simulink model "VSC"  (R2023a)
settings: Solver=FixedStepAuto  StartTime=0.0  StopTime=1  FixedStep=2e-6  RelTol=1e-3
InitFcn:
  | Ts=2e-6;
  | idref=20;
  | iqref=0;
  | Rs=3.75;
  | Ls=12e-3;
  | Lc=1.5e-3;
  | Us=100*sqrt(2);
  | omega_gn = 100*pi;
  | delta_ss=asin((omega_gn*Ls*idref+Rs*iqref)/Us);
  | zeta=0.5;
  | ts=0.1;
  | Kp=18.4/Us/ts;
  | Ki=43.32/Us/(zeta*ts)^2;
  | beta = 10*pi;
  | 
  | % Fault-time voltage dip
  | deltaV = 38.94*sqrt(2);
  | 
  | % Anti-windup parameters
  | k1=0;
  | k2=0;
  | % k1 = 5.9289;
  | % k2 = -7.7758;
  | % k2 = -k1 * Kp;
  | 
  | % performance-based activation of AW
  | % F = -353.46;
  | % F = -208.55;
  | F = 0;
undefined symbols (not defined in the file): Gp, Gq
libraries: spsControlledVoltageSourceLib x6, spsGroundLib x3, spsThreePhaseSeriesRLCBranchLib x3, eeGeneralControl x2, spsabctodq0Lib x2, spsPower3phInstantaneousLib x1, spsThreePhaseVIMeasurementLib x1, spsdq0toabcLib x1, spspowerguiLib x1
settings Model: Creator=Dell  LastModifiedBy=John Jackal
settings OptimizationCC: ReuseModelBlockBuffer=off
settings ModelReferenceCC: EnableRefExpFcnMdlSchedulingChecks=on

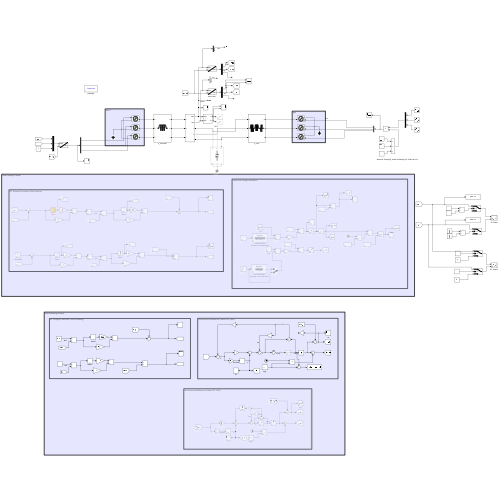
[thumbnail: Simulink's stored preview of the top-level diagram]
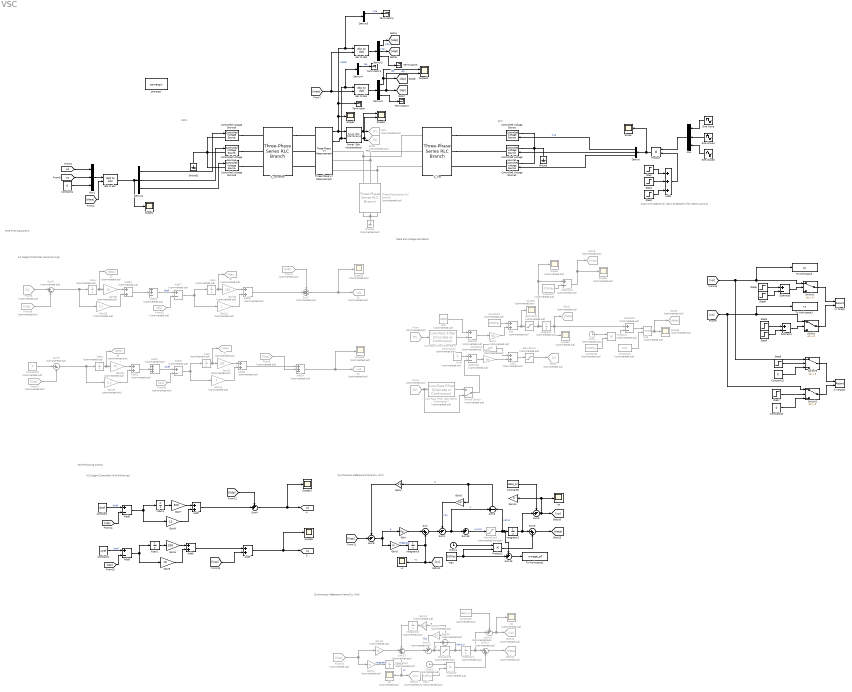
== system VSC ==
  note: Grid-Following Control
  note: Grid-Froming Control
  note: Synchronous-Reference Frame PLL (AW)
  note: AC Subgrid Controller (Grid-Following)
  note: PCC
  note: theta and voltage calculation
  note: start with 100sqrt(2), down to 60sqrt(2) for 100ms at t=1s
  note: grid
  note: VSC1
  note: AC Subgrid Controller (Grid-Forming)
  note: Synchronous-Reference Frame PLL (AW)
  "   21" : Goto  Commented=on  GotoTag=Xqaci  TagVisibility=global
  "   22" : Goto  Commented=on  GotoTag=Xdaci  TagVisibility=global
  "   23" : Goto  Commented=on  GotoTag=vq1  TagVisibility=global
  "   24" : Goto  Commented=on  GotoTag=vd1  TagVisibility=global
  "   25" : Goto  Commented=on  GotoTag=Xdacv  TagVisibility=global
  "   28" : Goto  Commented=on  GotoTag=Xqacv  TagVisibility=global
  Add{,1,22..23,25..26} (6 alike) : Sum  Commented=on
  Add19 : Sum  Commented=on  Inputs=++-
  Add2 : Sum  Inputs=+++
  Add21 : Sum  Commented=on  Inputs=+++
  Add24 : Sum  Commented=on  Inputs=++-
  Add27 : Sum  Commented=on  Inputs=+-
  Add28 : Sum  Commented=on  Inputs=+-
  Add5 : Sum
  Add6 : Sum
  Add7 : Sum
  Add8 : Sum  Inputs=+-
  Add9 : Sum  Inputs=+-
  Clock : Clock  Commented=on
  Clock1 : Clock
  Clock2 : Clock  Commented=on
  Constant : Constant  Value=idref
  Constant1 : Constant  Commented=on  Value=2*50*pi
  Constant10 : Constant  Value=0
  Constant11 : Constant  Value=0
  Constant2 : Constant  Value=iqref
  Constant20 : Constant  Commented=on  Value=0
  Constant3 : Constant  Commented=on  Value=100
  Constant4 : Constant  Value=0
  Constant5 : Constant  Commented=on  Value=2*50*pi
  Constant6 : Constant  Commented=on  Value=2*pi
  Constant7 : Constant  Commented=on  Value=2*50*pi
  Constant8 : Constant  Value=delta_ss
  Constant9 : Constant  Commented=on  Value=delta_ss
  Controlled Voltage Source{,1..5} (6 alike) : spsControlledVoltageSourceLib/Controlled Voltage Source  Initialize=on  Source_Type=AC  Amplitude=0  Phase=0  Frequency=0  Measurements=None
  Demux{,1..5} (6 alike) : Demux  Outputs=3
  From : From  Commented=on  GotoTag=P
  From1 : From  Commented=on  GotoTag=Q
  From16 : From  Commented=on  GotoTag=Uqp
  From39 : From  Commented=on  GotoTag=Uds
  From4 : From  Commented=on  GotoTag=Uds
  From47 : From  Commented=on  GotoTag=Uqs
  From5 : From  Commented=on  GotoTag=Uqs
  From6 : From  Commented=on  GotoTag=V
  From62 : From  Commented=on  GotoTag=ids
  From63 : From  Commented=on  GotoTag=iqs
  Gain : Gain  Gain=Kp
  Gain1 : Gain  Commented=on  Gain=Gp
  Gain10 : Gain  Commented=on  Gain=Kp
  Gain11 : Gain  Commented=on  Gain=Ki
  Gain12 : Gain  Commented=on  Gain=k1
  Gain13 : Gain  Commented=on  Gain=k2
  Gain14 : Gain  Gain=F
  Gain2 : Gain  Commented=on  Gain=Gq
  Gain29 : Gain  Commented=on  Gain=100
  Gain3 : Gain  Gain=Ki
  Gain30 : Gain  Commented=on  Gain=100
  Gain31 : Gain  Commented=on
  Gain35 : Gain  Commented=on  Gain=0.1
  Gain36 : Gain  Commented=on  Gain=10
  Gain37 : Gain  Commented=on  Gain=0.1
  Gain39 : Gain  Commented=on  Gain=10
  Gain4 : Gain  Gain=k1
  Gain41 : Gain  Commented=on
  Gain5 : Gain  Gain=k2
  Gain6 : Gain  Gain=500
  Gain7 : Gain  Gain=500
  Gain8 : Gain  Gain=10
  Gain9 : Gain  Gain=10
  Goto : Goto  Commented=on  GotoTag=P
  Goto1 : Goto  Commented=on  GotoTag=Q
  Goto12 : Goto  Commented=on  GotoTag=xp
  Goto14 : Goto  Commented=on  GotoTag=xc
  Goto15 : Goto  Commented=on  GotoTag=theta
  Goto2 : Goto  Commented=on  GotoTag=theta
  Goto3 : Goto  Commented=on  GotoTag=V
  Goto8 : Goto  Commented=on  GotoTag=delta
  Goto9 : Goto  Commented=on  GotoTag=omega
  Ground : spsGroundLib/Ground  LConnTagsString=a
  Ground1 : spsGroundLib/Ground  Commented=on  LConnTagsString=a
  Ground2 : spsGroundLib/Ground  LConnTagsString=a
  Integrator{,1,3..4} (4 alike) : Integrator  Commented=on
  Integrator2 : Integrator
  Integrator5 : Integrator
  Low-Pass Filter (Discrete or Continuous) : eeGeneralControl/Low-Pass Filter (Discrete or Continuous)  Commented=on  K=1  T=1/(2*pi*50)  B=inf  A=-inf  init_option=Inherited from block input  x0=0  Ts=-1
  Low-Pass Filter (Discrete or Continuous)1 : eeGeneralControl/Low-Pass Filter (Discrete or Continuous)  Commented=on  K=1  T=1/(2*pi*0.1)  B=inf  A=-inf  init_option=Inherited from block input  x0=0  Ts=-1
  Manual Switch : ManualSwitch  Commented=on  CurrentSetting=0
  Mod : Math  Commented=on  Operator=mod
  Mux : Mux  Inputs=3
  Mux1 : Mux  Inputs=3
  "Power (3ph, Instantaneous)" : spsPower3phInstantaneousLib/Power (3ph, Instantaneous)
  Pref : Constant  Commented=on  Value=2000
  Product : Product
  Product1 : Product  Commented=on
  Product2 : Product
  Product3 : Product  Commented=on
  Qref : Constant  Commented=on  Value=0
  Saturation : Saturate  Commented=on  UpperLimit=51*2*pi  LowerLimit=49*2*pi
  Saturation1 : Saturate  Commented=on  UpperLimit=150  LowerLimit=50
  Saturation2 : Saturate  Commented=through  UpperLimit=beta  LowerLimit=-beta
  Saturation3 : Saturate  Commented=on  UpperLimit=10*pi  LowerLimit=-10*pi
  Scope{,1..2,9..10} (5 alike) : Scope
  Scope11 : Scope  NumInputPorts=2
  Scope{4..8,18,25} (7 alike) : Scope  Commented=on
  Scope3 : Scope  NumInputPorts=2
  Sine Wave : Sin  Frequency=50*2*pi  SampleTime=Ts
  Sine Wave1 : Sin  Frequency=50*2*pi  Phase=-2/3*pi  SampleTime=Ts
  Sine Wave2 : Sin  Frequency=50*2*pi  Phase=2/3*pi  SampleTime=Ts
  Step : Step  Time=0  Before=Us  After=Us  SampleTime=0
  Step1 : Step  Time=0.1  After=-deltaV  SampleTime=0
  Step2 : Step  Time=0.2  After=deltaV  SampleTime=0
  Step3 : Step  Time=0  SampleTime=0
  Step4 : Step  SampleTime=0
  Step5 : Step  Time=0  SampleTime=0
  Step6 : Step  SampleTime=0
  Step7 : Step  Time=3  SampleTime=0
  Step9 : Step  Time=3  SampleTime=0
  Subtract{,1..3} (4 alike) : Sum  Commented=on  Inputs=+-
  Subtract4 : Sum  Inputs=+-
  Subtract5 : Sum  Inputs=+-
  Sum : Sum  Inputs=|++
  Sum1 : Sum  Inputs=-+|
  Sum10 : Sum  Commented=on  Inputs=-++
  Sum11 : Sum  Commented=on  Inputs=-+|
  Sum12 : Sum  Commented=on  Inputs=+-
  Sum13 : Sum  Commented=on  Inputs=|++
  Sum14 : Sum  Commented=on  Inputs=-+|
  Sum15 : Sum  Inputs=++|
  Sum16 : Sum  Inputs=++|
  Sum2 : Sum  Inputs=+-
  Sum3 : Sum  Inputs=|++
  Sum4 : Sum  Inputs=++|
  Sum5 : Sum  Inputs=-+|
  Sum6 : Sum  Commented=on  Inputs=|+-
  Sum7 : Sum  Commented=on  Inputs=+++
  Sum8 : Sum  Inputs=-+|
  Sum9 : Sum  Commented=on  Inputs=|+-
  Switch{,1..3} (4 alike) : Switch  Criteria=u2 > Threshold  SaturateOnIntegerOverflow=off  InputSameDT=off
  Terminator{,1..4} (5 alike) : Terminator
  Three-Phase Series RLC Branch1 : spsThreePhaseSeriesRLCBranchLib/Three-Phase Series RLC Branch  Commented=on  LConnTagsString=A|B|C  RConnTagsString=A|B|C  BranchType=C  Resistance=1  Inductance=1e-3  Capacitance=20e-6  Measurements=None
  Three-Phase V-I Measurement : spsThreePhaseVIMeasurementLib/Three-Phase V-I Measurement  VoltageMeasurement=phase-to-ground  SetLabelV=off  LabelV=Vabc  Vpu=off  VpuLL=off  CurrentMeasurement=yes  SetLabelI=off  LabelI=Iabc  Ipu=off  Pbase=100e6  Vbase=500e3  OutputType=Complex  PhasorSimulation=off  PSBequivalent=0
  To Workspace : ToWorkspace  VariableName=xp  SampleTime=-1
  To Workspace1 : ToWorkspace  VariableName=xc  SampleTime=-1
  To Workspace2 : ToWorkspace  VariableName=omega_pll  SampleTime=-1
  XY Graph : Record  RecordToWorkspace=on  FileSettingsInternal="{\"entries\":[{\"content\":{\"excelSettings\":{\"content\":{},\"type\":\"Streamout.ExcelSettings\"}},\"type\":\"Streamout.FileSettingStorage\",\"uuid\":\"61cb4bfb-05d6-417b-9b14-40baebda5446\"}],\"packageUris\":[\"http://schema.mathworks.com/mf0/streamout_blocks/R2020a\"],\"version\":\"1.0\"}"  Layout=[1 1]  SignalsInternal="{\"entries\":[{\"content\":{\"signals\":[{\"content\":{\"blockPath\":[\"VSC/XY Graph\"],\"dimensions\":[1],\"domain\":\"VSC/XY Graph\",\"lineColor\":\"#a2142f\",\"plots\":[1],\"port\":1,\"sid\":[\"\"],\"signalID\":410486,\"signalName\":\"Switch1\"},\"type\":\"RecordBlkView.Signal\",\"uuid\":\"486c21a0-9f22-4725-bac4-aafadb3d172d\"},{\"content\":{\"blockPath\":[\"VSC/XY Graph\"],\"dimensions\":[1],\"domain\":\"VSC/XY Graph\",\"lineColor\":\"#139fff\",\"plots\":[1],\"port\":2,\"sid\":[\"\"],\"signalID\":410490,\"signalName\":\"Switch\"},\"type\":\"RecordBlkView.Signal\",\"uuid\":\"b45c9456-2913-48ec-872b-2d38d1e96725\"}]},\"type\":\"RecordBlkView.InputSignals\",\"uuid\":\"3a20c26a-c753-4ebd-9899-0a237facdabc\"}],\"packageUris\":[\"http://schema.mathworks.com/mf0/streamout_blocks/R2020a\"],\"version\":\"1.0\"}"  VisualizationBindings="{\"xyplotplugin\":{\"info\":[{\"series\":[{\"bindingParametersList\":[{\"parameter\":\"X-Axis\",\"signalID\":410486,\"signalName\":\"Switch1\"},{\"parameter\":\"Y-Axis\",\"signalID\":410490,\"signalName\":\"Switch\"}],\"seriesID\":23615}],\"subplotID\":1}]}}"  CompatibilityTag=XY
  XY Graph1 : Record  FileSettingsInternal="{\"entries\":[{\"content\":{\"excelSettings\":{\"content\":{},\"type\":\"Streamout.ExcelSettings\"}},\"type\":\"Streamout.FileSettingStorage\",\"uuid\":\"121f3693-127c-40a0-ad6a-a4d3c19ad6c3\"}],\"packageUris\":[\"http://schema.mathworks.com/mf0/streamout_blocks/R2020a\"],\"version\":\"1.0\"}"  Layout=[1 1]  SignalsInternal="{\"entries\":[{\"content\":{\"signals\":[{\"content\":{\"blockPath\":[\"VSC/XY Graph1\"],\"dimensions\":[1],\"domain\":\"VSC/XY Graph1\",\"lineColor\":\"#a2142f\",\"plots\":[1],\"port\":1,\"sid\":[\"\"],\"signalID\":410494,\"signalName\":\"Switch3\"},\"type\":\"RecordBlkView.Signal\",\"uuid\":\"372b1ac4-6cda-481d-8315-b179240ae1fd\"},{\"content\":{\"blockPath\":[\"VSC/XY Graph1\"],\"dimensions\":[1],\"domain\":\"VSC/XY Graph1\",\"lineColor\":\"#139fff\",\"plots\":[1],\"port\":2,\"sid\":[\"\"],\"signalID\":410498,\"signalName\":\"Switch2\"},\"type\":\"RecordBlkView.Signal\",\"uuid\":\"0dfc1476-e637-47cc-b005-821a066936e3\"}]},\"type\":\"RecordBlkView.InputSignals\",\"uuid\":\"1970ed3a-d7d9-4a85-a3e3-02939245d4e1\"}],\"packageUris\":[\"http://schema.mathworks.com/mf0/streamout_blocks/R2020a\"],\"version\":\"1.0\"}"  VisualizationBindings="{\"xyplotplugin\":{\"info\":[{\"series\":[{\"bindingParametersList\":[{\"parameter\":\"X-Axis\",\"signalID\":410494,\"signalName\":\"Switch3\"},{\"parameter\":\"Y-Axis\",\"signalID\":410498,\"signalName\":\"Switch2\"}],\"seriesID\":51744}],\"subplotID\":1}]}}"  CompatibilityTag=XY
  Xdaci : Integrator  Commented=on  InitialCondition=0.01  IgnoreLimit=on
  Xdaci1 : Integrator  InitialCondition=0.01  IgnoreLimit=on
  Xdacv : Integrator  Commented=on  InitialCondition=1.3  IgnoreLimit=on
  Xqaci : Integrator  Commented=on  InitialCondition=0.067  IgnoreLimit=on
  Xqaci1 : Integrator  InitialCondition=0.067  IgnoreLimit=on
  Xqacv : Integrator  Commented=on  InitialCondition=-0.2  IgnoreLimit=on
  Z_converter : spsThreePhaseSeriesRLCBranchLib/Three-Phase Series RLC Branch  LConnTagsString=A|B|C  RConnTagsString=A|B|C  BranchType=L  Resistance=1  Inductance=Lc  Capacitance=1e-6  Measurements=None
  Z_line : spsThreePhaseSeriesRLCBranchLib/Three-Phase Series RLC Branch  LConnTagsString=A|B|C  RConnTagsString=A|B|C  BranchType=RLC  Resistance=Rs  Inductance=Ls  Capacitance=0  Measurements=None
  abc to dq0 : spsabctodq0Lib/abc to dq0  Alignment=90 degrees behind phase A axis
  abc to dq1 : spsabctodq0Lib/abc to dq0  Alignment=90 degrees behind phase A axis
  dq0 to abc : spsdq0toabcLib/dq0 to abc  Alignment=90 degrees behind phase A axis
  powergui : spspowerguiLib/powergui  Priority=1  SimulationMode=Continuous  SampleTime=2e-6  frequency=60  Iterations=50  frequencyindice=0  Pbase=100e6  ErrMax=1e-4  UnitsV=kV  UnitsW=MW  buscounter=0  FunctionMessages=off  echomessages=off  EnableUseOfTLC=off  CurrentSourceSwitches=off  DisableSnubberDevices=off  DisableRonSwitches=off  DisableVfSwitches=off  DisplayEquations=off  AutomaticDiscreteSolvers=off  SolverType=Tustin/Backward Euler (TBE)  Interpol=off  ExternalGateDelay=off  methode=off  Ts=100  x0status=blocks  SPID=on  SwTol=0  HookPort=off  NonlinearTolerance=1e-4  nMaxIteration=100  ContinueOnMaxIteration=off  RestoreLinks=warning  ResistiveCurrentMeasurement=off  Frange=[0:2:500]  Ylog=off  Xlog=on  ShowGrid=off  save=off  variable=ZData  structure=0  ZoomFFT=off  StartTime=0.0  cycles=1  DisplayStyle=1  fundamental=60  FreqAxis=off  MaxFrequency=1000  frequencyindicesteady=1  RmsSteady=1  display=off
  wgn : Constant  Value=100*pi
  wgn1 : Constant  Commented=on  Value=100*pi
  xc : Scope
  xc1 : Scope  Commented=on
  xp : Scope
  xp1 : Scope  Commented=on
  tag scope: vd=global, vq=global
  wires:
  Demux/1 -> Controlled Voltage Source/1  "Vsa"
  Demux/3 -> Controlled Voltage Source2/1
  Demux/2 -> Controlled Voltage Source1/1
  Sine Wave/1 -> Mux/1
  Sine Wave1/1 -> Mux/2
  Sine Wave2/1 -> Mux/3
  Mux/1 -> Product/1
  Product/1 -> Scope/1, Demux/1
  Three-Phase V-I Measurement/1 -> Terminator/1, Demux5/1, abc to dq0/1, Scope2/1, "Power (3ph, Instantaneous)"/1  "Vpabc"
  Three-Phase V-I Measurement/2 -> Demux4/1, abc to dq1/1, "Power (3ph, Instantaneous)"/2
  "Power (3ph, Instantaneous)"/1 -> Scope3/1, Goto/1
  "Power (3ph, Instantaneous)"/2 -> Scope3/2, Goto1/1
  Pref/1 -> Subtract/1
  From/1 -> Low-Pass Filter (Discrete or Continuous)/1
  Subtract/1 -> Gain1/1
  Gain1/1 -> Add/2
  Constant1/1 -> Add/1
  Add/1 -> Scope5/1, Saturation/1
  Integrator/1 -> Goto2/1, Subtract2/1, Scope4/1
  Add1/1 -> Saturation1/1
  Constant3/1 -> Add1/1
  Gain2/1 -> Add1/2
  Subtract1/1 -> Gain2/1
  From1/1 -> Manual Switch/2, Low-Pass Filter (Discrete or Continuous)1/1
  Qref/1 -> Subtract1/1
  dq0 to abc/1 -> Scope1/1, Demux1/1
  Demux1/1 -> Controlled Voltage Source5/1
  Demux1/2 -> Controlled Voltage Source4/1
  Demux1/3 -> Controlled Voltage Source3/1
  Saturation1/1 -> Goto3/1
  From62/1 -> Add27/2
  Xqaci/1 -> "   21"/1, Gain29/1
  Add27/1 -> Gain31/1, Xdaci/1
  Add21/1 -> Add28/1  "iqref"
  Sum6/1 -> Gain35/1, Xdacv/1
  Add24/1 -> "   23"/1, Scope18/1
  From39/1 -> Sum6/2
  Add28/1 -> Xqaci/1, Gain41/1
  Gain31/1 -> Add26/2
  Gain41/1 -> Add25/2
  From6/1 -> Sum6/1
  Gain39/1 -> Add22/1
  Constant20/1 -> Sum9/1
  Gain37/1 -> Add22/2
  Add22/1 -> Add21/2
  Gain30/1 -> Add26/1
  Gain36/1 -> Add23/1
  Gain29/1 -> Add25/1
  Add23/1 -> Add19/2
  Gain35/1 -> Add23/2
  From47/1 -> Sum9/2
  Xdacv/1 -> "   25"/1, Gain36/1
  Sum7/1 -> "   24"/1, Scope25/1
  Xdaci/1 -> Gain30/1, "   22"/1
  Add19/1 -> Add27/1  "idref"
  From63/1 -> Add28/2
  Add25/1 -> Add24/1
  From5/1 -> Add24/2
  From4/1 -> Sum7/1
  Add26/1 -> Sum7/2
  Sum9/1 -> Xqacv/1, Gain37/1
  Xqacv/1 -> "   28"/1, Gain39/1
  [theta] -> abc to dq0/2, abc to dq1/2
  abc to dq0/1 -> Demux2/1
  Demux2/1 -> [Udp]  "Vdp"
  Demux2/2 -> [Uqp]  "Vqp"
  Demux3/2 -> Scope11/2, [iqp]  "iqp"
  Demux3/1 -> Scope11/1, [idp]  "idp"
  abc to dq1/1 -> Demux3/1
  [theta] -> dq0 to abc/2
  Mux1/1 -> dq0 to abc/1
  [vd] -> Mux1/1
  [vq] -> Mux1/2
  Constant4/1 -> Mux1/3
  Add2/1 -> Product/2
  Step/1 -> Add2/1
  Step1/1 -> Add2/2
  Step2/1 -> Add2/3
  Clock/1 -> Product1/1
  Constant5/1 -> Product1/2
  Product1/1 -> Subtract2/2
  Subtract2/1 -> Mod/1
  Constant6/1 -> Mod/2
  Mod/1 -> Goto8/1, Scope6/1
  Saturation/1 -> Subtract3/1, Scope7/1, Integrator/1
  Constant7/1 -> Subtract3/2
  Subtract3/1 -> Scope8/1, Goto9/1
  Switch/1 -> XY Graph/2
  Step3/1 -> Subtract4/1
  Subtract4/1 -> Switch/2
  Step4/1 -> Subtract4/2
  Step6/1 -> Subtract5/2
  Subtract5/1 -> Switch1/2
  Step5/1 -> Subtract5/1
  Switch1/1 -> XY Graph/1
  Constant11/1 -> Switch3/3
  Step9/1 -> Switch3/2
  [xp] -> To Workspace/1, Switch1/1, Switch3/1
  [xc] -> To Workspace1/1, Switch/1, Switch2/1
  Step7/1 -> Switch2/2
  Constant10/1 -> Switch2/3
  Switch3/1 -> XY Graph1/1
  Switch2/1 -> XY Graph1/2
  Low-Pass Filter (Discrete or Continuous)/1 -> Subtract/2
  Low-Pass Filter (Discrete or Continuous)1/1 -> Manual Switch/1
  Manual Switch/1 -> Subtract1/2
  Sum1/1 -> Sum16/2, Sum2/1  "u"
  Saturation2/1 -> Sum2/2, Sum15/1, Integrator2/1  "sat(u)"
  Sum/1 -> Sum1/2
  Gain3/1 -> Integrator5/1  "integrator"
  Sum2/1 -> Gain5/1, Gain4/1  "q"
  Gain5/1 -> Sum1/1  "k2q"
  Integrator2/1 -> Sum5/2, Sum3/1
  Sum3/1 -> [theta]
  Clock1/1 -> Product2/1
  wgn/1 -> Sum15/2, Product2/2
  Product2/1 -> Sum3/2
  Gain6/1 -> Add6/1
  Add5/1 -> [vq], Scope9/1
  Sum4/1 -> [vd], Scope10/1
  Add6/1 -> Add5/1
  [Udp] -> Sum4/1
  Gain8/1 -> Add7/2
  Constant/1 -> Add8/1  "idref"
  Add7/1 -> Sum4/2
  Constant2/1 -> Add9/1  "iqref"
  Gain9/1 -> Add6/2
  Add9/1 -> Xqaci1/1, Gain9/1
  Gain7/1 -> Add7/1
  Xdaci1/1 -> Gain7/1
  [Uqp] -> Add5/2
  Add8/1 -> Gain8/1, Xdaci1/1
  [iqp] -> Add9/2
  Xqaci1/1 -> Gain6/1
  [idp] -> Add8/2
  Demux3/3 -> Terminator2/1
  Demux2/3 -> Terminator3/1
  Demux5/1 -> Terminator4/1  "Vpa"
  Demux4/1 -> Terminator1/1  "Ipa"
  Constant8/1 -> Sum5/1
  Sum5/1 -> xp/1, Gain14/1, [xp]
  Gain/1 -> Sum/1
  Integrator5/1 -> xc/1, [xc], Sum/2  "xc"
  [Uqp] -> Sum8/2
  Sum8/1 -> Gain3/1, Gain/1  "e"
  Gain4/1 -> Sum8/1
  Constant9/1 -> Sum14/1
  From16/1 -> Gain11/1, Gain10/1
  Sum14/1 -> xp1/1, Goto12/1
  Gain13/1 -> Sum11/1  "k2q"
  Clock2/1 -> Product3/1
  wgn1/1 -> Product3/2
  Product3/1 -> Sum13/2
  Sum12/1 -> Gain12/1, Gain13/1  "q"
  Sum13/1 -> Goto15/1
  Gain11/1 -> Integrator3/1  "integrator"
  Integrator1/1 -> Sum14/2, Sum13/1
  Sum10/1 -> Sum11/2
  Saturation3/1 -> Sum12/2, Integrator1/1  "\\hat{u}"
  Sum11/1 -> Sum12/1, Saturation3/1  "u"
  Gain12/1 -> Integrator4/1
  Integrator4/1 -> Sum10/1
  Gain10/1 -> Sum10/2
  Integrator3/1 -> xc1/1, Goto14/1, Sum10/3  "xc"
  Sum15/1 -> To Workspace2/1
  Sum16/1 -> Saturation2/1  "u+Fxp"
  connections:
  Controlled Voltage Source/LConn1 -- Controlled Voltage Source2/LConn1 -- Controlled Voltage Source1/LConn1 -- Ground/LConn1
  Z_line/RConn2 -- Controlled Voltage Source1/RConn1
  Z_line/RConn1 -- Controlled Voltage Source/RConn1
  Controlled Voltage Source2/RConn1 -- Z_line/RConn3
  Three-Phase Series RLC Branch1/LConn1 -- Three-Phase V-I Measurement/RConn1 -- Z_line/LConn1
  Three-Phase Series RLC Branch1/LConn3 -- Z_line/LConn3 -- Three-Phase V-I Measurement/RConn3
  Three-Phase Series RLC Branch1/LConn2 -- Z_line/LConn2 -- Three-Phase V-I Measurement/RConn2
  Ground1/LConn1 -- Three-Phase Series RLC Branch1/RConn3 -- Three-Phase Series RLC Branch1/RConn1 -- Three-Phase Series RLC Branch1/RConn2
  Controlled Voltage Source5/LConn1 -- Ground2/LConn1 -- Controlled Voltage Source3/LConn1 -- Controlled Voltage Source4/LConn1
  Controlled Voltage Source5/RConn1 -- Z_converter/LConn1
  Controlled Voltage Source4/RConn1 -- Z_converter/LConn2
  Controlled Voltage Source3/RConn1 -- Z_converter/LConn3
  Z_converter/RConn1 -- Three-Phase V-I Measurement/LConn1
  Three-Phase V-I Measurement/LConn2 -- Z_converter/RConn2
  Three-Phase V-I Measurement/LConn3 -- Z_converter/RConn3
